simulink model "adaptive_cruise_control_model"  (R2018a)
settings: Solver=ode23t  StartTime=0.0  StopTime=150  MaxStep=0.01  RelTol=1e-3
values from neighbouring files (symbols this model uses):
  ddefault = 5    [linearized_parameters.m]
  K = 0.07536    [linearized_parameters.m]
  rw = 0.3    [linearized_parameters.m]
  tlag = 3    [linearized_parameters.m]
undefined symbols (not defined in the file or in its folder): sigbuilder_block
libraries: simulink x7, dspsigops x1
settings Model: EnablePacing=on  Creator=Saurabh Suman  LastModifiedBy=Saurabh Suman

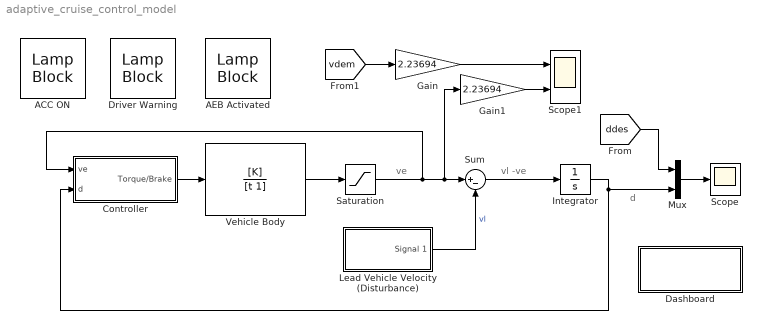
== system adaptive_cruise_control_model ==
  note: d
  note: vl -ve
  note: ve
  ACC ON : LampBlock  WebBlockId=122
  AEB Activated : LampBlock  WebBlockId=120
  Controller : Subsystem
  Dashboard : Subsystem
  Driver Warning : LampBlock  WebBlockId=121
  Gain : Gain  Gain=2.23694
  Gain1 : Gain  Gain=2.23694
  Integrator : Integrator  InitialCondition=100
  Lead Vehicle Velocity (Disturbance) : Subsystem  Tag=STV Subsys  LoadFcn=sigbuilder_block('load');  StartFcn=sigbuilder_block('start');  StopFcn=sigbuilder_block('stop');  ClipboardFcn=sigbuilder_block('clipboard');  mask(Sigbuilder block){tuvar=[0:10]}
      mask help: Simulink:masks:SigbuilderBlock_MD
      mask init:
      | if ~strcmp(get_param(bdroot(gcbh),'SimulationStatus'),'stopped') tuvar = sigbuilder_block('maskInit'); end
      settings: CopyFcn=sigbuilder_block('copy');  DeleteFcn=sigbuilder_block('delete');  ModelCloseFcn=sigbuilder_block('modelClose');  PreSaveFcn=sigbuilder_block('preSave');  PauseFcn=sigbuilder_block('pause');  ContinueFcn=sigbuilder_block('continue');  NameChangeFcn=sigbuilder_block('namechange');  OpenFcn=sigbuilder_block('open',[456.6 167.4 550.8 400.2 ]);  CloseFcn=sigbuilder_block('close');
      mask Display: plot(0, 0, 100, 100,[2, 2, 32, 32, 2], [68, 8, 8, 68, 68],[32, 2], [38, 38], [32, 19, 2],[53, 60, 44], [32, 17, 17, 2],[16, 16, 31, 31]);txt = getActiveGroup(gcbh);text(2, 100, txt,'verticalAlignment', 'top');
  Mux : Mux  Inputs=2
  Saturation : Saturate  UpperLimit=Inf  LowerLimit=0  ZeroCross=off
  Scope : Scope
  Scope1 : Scope  NumInputPorts=2
  Sum : Sum  Inputs=|+-
  Vehicle Body : TransferFcn  Numerator=[K]  Denominator=[t 1]
  wires:
  Lead Vehicle Velocity (Disturbance)/1(Signal 1) -> Sum/2  "vl"
  Saturation/1 -> Controller/1(ve), Gain1/1, Sum/1
  Vehicle Body/1 -> Saturation/1
  Controller/1(Torque/Brake) -> Vehicle Body/1
  Sum/1 -> Integrator/1
  Integrator/1 -> Mux/2, Controller/2(d)
  [ddes] -> Mux/1
  Mux/1 -> Scope/1
  [vdem] -> Gain/1
  Gain/1 -> Scope1/1
  Gain1/1 -> Scope1/2

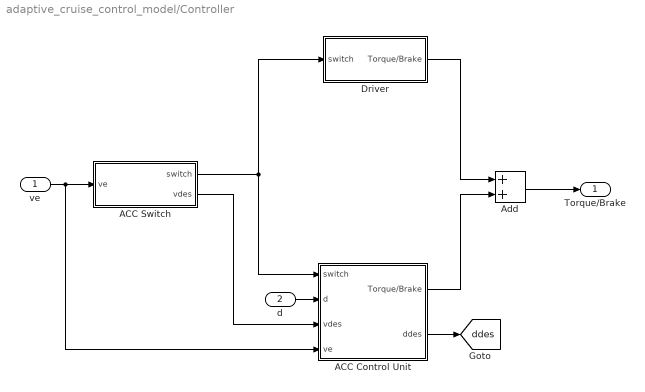
== system adaptive_cruise_control_model/Controller ==
  ve : Inport
  d : Inport  Port=2
  ACC Control Unit : Subsystem
  ACC Switch : Subsystem
  Add : Sum
  Driver : Subsystem
  Torque/Brake : Outport
  tag scope: ddes=global
  wires:
  ve/1 -> ACC Control Unit/4(ve), ACC Switch/1(ve)
  d/1 -> ACC Control Unit/2(d)
  ACC Switch/1(switch) -> Driver/1(switch), ACC Control Unit/1(switch)
  ACC Switch/2(vdes) -> ACC Control Unit/3(vdes)
  ACC Control Unit/1(Torque/Brake) -> Add/2
  Driver/1(Torque/Brake) -> Add/1
  Add/1 -> Torque/Brake/1
  ACC Control Unit/2(ddes) -> [ddes]

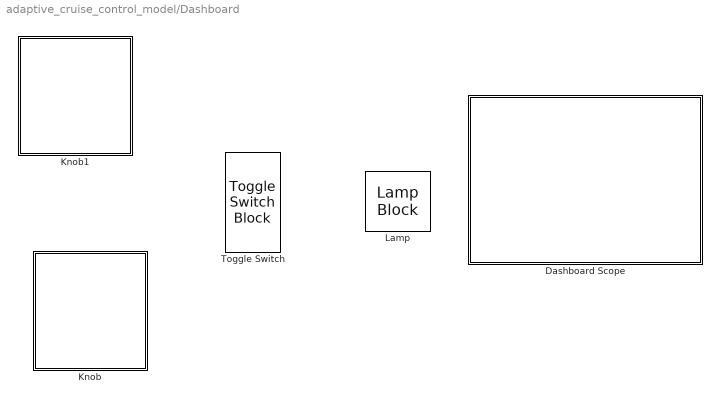
== system adaptive_cruise_control_model/Dashboard ==
  Dashboard Scope : Subsystem  DialogController=hmiCreateDDGDialog  IsWebBlock=on  mask(MWDashboardBlock){webBlockId=a9cadf37-32fc-4d88-93af-27b178824d04, webBlockType=sdiscope, ShowInitialText=on, HMISrcModelName=adaptive_cruise_control_model}
      mask prompts: webBlockId "WebBlock Id"; webBlockType "WebBlock Type"; HMISrcModelName "Source Model"
      mask help: SimulinkHMI:dialogs:HMIScopeDialogDesc
      mask Help: helpview([docroot '/mapfiles/simulink.map'], 'hmi_scope')
      mask Display:
      | if strcmp(get_param(bdroot(gcb),'BlockDiagramType'), 'library')
      |     image([(matlabroot) '/toolbox/simulink/hmi/icons/DashboardScope.png']);
      | end
  Knob : Subsystem  DialogController=hmiCreateDDGDialog  IsWebBlock=on  mask(MWDashboardBlock){webBlockId=72363b14-a3cf-4823-9712-4e9a4279af6e, webBlockType=continuousknob, ShowInLibBrowser=on, ShowInitialText=on, HMISrcModelName=adaptive_cruise_control_model}
      mask prompts: webBlockId "WebBlock Id"; webBlockType "WebBlock Type"; HMISrcModelName "Source Model"
      mask help: SimulinkHMI:dialogs:ContinuousKnobDialogDesc
      mask Help: helpview([docroot '/mapfiles/simulink.map'], 'hmi_knob')
      mask Display:
      | if strcmp(get_param(bdroot(gcb),'BlockDiagramType'), 'library')
      |     image([(matlabroot) '/toolbox/simulink/hmi/icons/ContinuousKnob.png']);
      | end
  Knob1 : Subsystem  DialogController=hmiCreateDDGDialog  IsWebBlock=on  mask(MWDashboardBlock){webBlockId=54317ec1-8d0a-43bc-8178-3813509fb264, webBlockType=continuousknob, ShowInLibBrowser=on, ShowInitialText=on, HMISrcModelName=adaptive_cruise_control_model}
      mask prompts: webBlockId "WebBlock Id"; webBlockType "WebBlock Type"; HMISrcModelName "Source Model"
      mask help: SimulinkHMI:dialogs:ContinuousKnobDialogDesc
      mask Help: helpview([docroot '/mapfiles/simulink.map'], 'hmi_knob')
      mask Display:
      | if strcmp(get_param(bdroot(gcb),'BlockDiagramType'), 'library')
      |     image([(matlabroot) '/toolbox/simulink/hmi/icons/ContinuousKnob.png']);
      | end
  Lamp : LampBlock  WebBlockId=128
  Toggle Switch : ToggleSwitchBlock  WebBlockId=129
      settings: Values={{'Off', 'On'}, [0 1]}

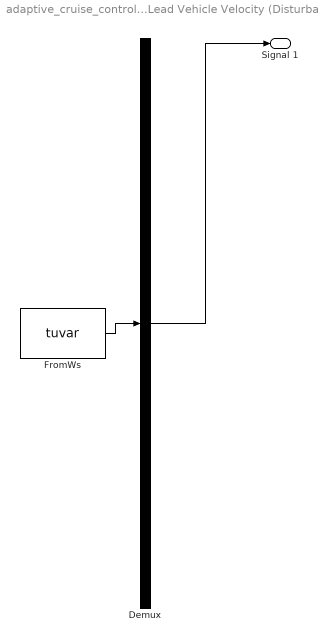
== system adaptive_cruise_control_model/Lead Vehicle Velocity (Disturbance) ==
  Demux : Demux  Tag=STV Demux  Outputs=1
  FromWs : FromWorkspace  Tag=STV FromWs  VariableName=tuvar  SampleTime=0
      SigBuilderData=|
      | common.afterFinalStr = 'Extrapolate'
      | common.sampleTime = 0
      | dataSet(1).timeRange = [0 150]
      | dataSet(1).name = 'Scenario 1'
      | dataSet(2).timeRange = [0 150]
      | dataSet(2).name = 'Scenario 2'
      | dataSet(3).timeRange = [0 150]
      | dataSet(3).name = 'Scenario 3'
      | dataSet(4).timeRange = [0 150]
      | dataSet(4).name = 'Scenario 4'
      | sbobj.Groups(1).Name = 'Scenario 1'
      | sbobj.Groups(1).Signals.Name = 'Signal 1'
      | sbobj.Groups(1).Signals.XData = [0 150]
      | sbobj.Groups(1).Signals.YData = [40 40]
      | sbobj.Groups(1).TimeRange = [0 150]
      | sbobj.Groups(2).Name = 'Scenario 2'
      | sbobj.Groups(2).Signals.Name = 'Signal 1'
      | sbobj.Groups(2).Signals.XData = [0 30 70 80 100 150]
      | sbobj.Groups(2).Signals.YData = [25 25 15 15 30 30]
      | sbobj.Groups(2).TimeRange = [0 150]
      | sbobj.Groups(3).Name = 'Scenario 3'
      | sbobj.Groups(3).Signals.Name = 'Signal 1'
      | sbobj.Groups(3).Signals.XData = [0 30 70 80 100 150]
      | sbobj.Groups(3).Signals.YData = [25 25 15 15 25 25]
      | sbobj.Groups(3).TimeRange = [0 150]
      | sbobj.Groups(4).Name = 'Scenario 4'
      | sbobj.Groups(4).Signals.Name = 'Signal 1'
      | sbobj.Groups(4).Signals.XData = [0 30 70 80 100 150]
      | sbobj.Groups(4).Signals.YData = [25 25 0 0 25 25]
      | sbobj.Groups(4).TimeRange = [0 150]
  Signal 1 : Outport  Tag=STV Outport
  wires:
  Demux/1 -> Signal 1/1
  FromWs/1 -> Demux/1

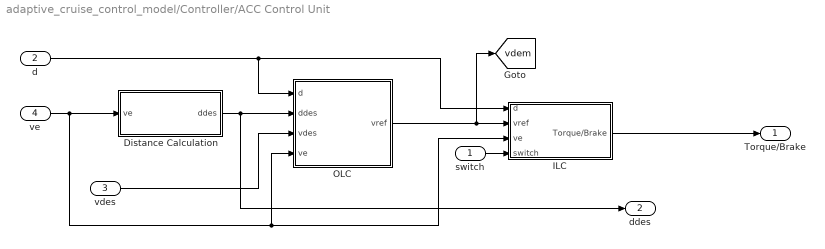
== system adaptive_cruise_control_model/Controller/ACC Control Unit ==
  switch : Inport
  d : Inport  Port=2
  vdes : Inport  Port=3
  ve : Inport  Port=4
  Distance Calculation : Subsystem
  ILC : Subsystem
  OLC : Subsystem
  Torque/Brake : Outport
  ddes : Outport  Port=2
  tag scope: vdem=global
  wires:
  OLC/1(vref) -> [vdem], ILC/2(vref)
  d/1 -> ILC/1(d), OLC/1(d)
  ve/1 -> ILC/3(ve), OLC/4(ve), Distance Calculation/1(ve)
  Distance Calculation/1(ddes) -> ddes/1, OLC/2(ddes)
  vdes/1 -> OLC/3(vdes)
  switch/1 -> ILC/4(switch)
  ILC/1(Torque/Brake) -> Torque/Brake/1

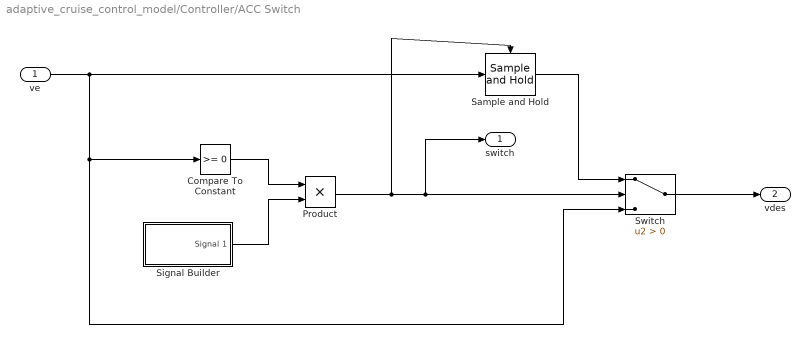
== system adaptive_cruise_control_model/Controller/ACC Switch ==
  ve : Inport
  Compare To Constant : simulink/Logic and Bit Operations/Compare To Constant  relop=>=  const=0  OutDataTypeStr=boolean
  Product : Product
  Sample and Hold : dspsigops/Sample and Hold  trig=Rising edge  initCond=0  latchinput=off
  Signal Builder : Subsystem  Tag=STV Subsys  LoadFcn=sigbuilder_block('load');  StartFcn=sigbuilder_block('start');  StopFcn=sigbuilder_block('stop');  ClipboardFcn=sigbuilder_block('clipboard');  mask(Sigbuilder block){tuvar=[0:10]}
      mask help: Simulink:masks:SigbuilderBlock_MD
      mask init:
      | if ~strcmp(get_param(bdroot(gcbh),'SimulationStatus'),'stopped') tuvar = sigbuilder_block('maskInit'); end
      settings: CopyFcn=sigbuilder_block('copy');  DeleteFcn=sigbuilder_block('delete');  ModelCloseFcn=sigbuilder_block('modelClose');  PreSaveFcn=sigbuilder_block('preSave');  PauseFcn=sigbuilder_block('pause');  ContinueFcn=sigbuilder_block('continue');  NameChangeFcn=sigbuilder_block('namechange');  OpenFcn=sigbuilder_block('open',[453.6 160.2 550.8 400.2 ]);  CloseFcn=sigbuilder_block('close');
      mask Display: plot(0, 0, 100, 100,[2, 2, 32, 32, 2], [68, 8, 8, 68, 68],[32, 2], [38, 38], [32, 19, 2],[53, 60, 44], [32, 17, 17, 2],[16, 16, 31, 31]);txt = getActiveGroup(gcbh);text(2, 100, txt,'verticalAlignment', 'top');
  Switch : Switch  Criteria=u2 > Threshold
  switch : Outport
  vdes : Outport  Port=2
  wires:
  Sample and Hold/1 -> Switch/1
  Switch/1 -> vdes/1
  Compare To Constant/1 -> Product/1
  Signal Builder/1(Signal 1) -> Product/2
  ve/1 -> Compare To Constant/1, Switch/3, Sample and Hold/1
  Product/1 -> Sample and Hold/Trigger, switch/1, Switch/2

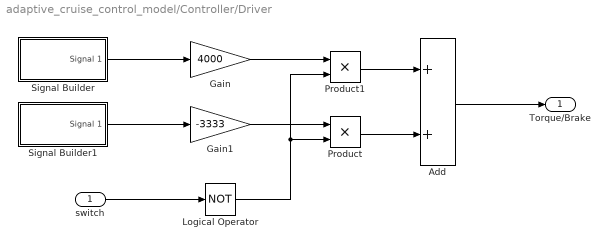
== system adaptive_cruise_control_model/Controller/Driver ==
  switch : Inport
  Add : Sum
  Gain : Gain  Gain=4000
  Gain1 : Gain  Gain=-3333
  Logical Operator : Logic  Operator=NOT  AllPortsSameDT=off  OutDataTypeStr=boolean
  Product : Product
  Product1 : Product
  Signal Builder : Subsystem  Tag=STV Subsys  LoadFcn=sigbuilder_block('load');  StartFcn=sigbuilder_block('start');  StopFcn=sigbuilder_block('stop');  ClipboardFcn=sigbuilder_block('clipboard');  mask(Sigbuilder block){tuvar=[0:10]}
      mask help: Simulink:masks:SigbuilderBlock_MD
      mask init:
      | if ~strcmp(get_param(bdroot(gcbh),'SimulationStatus'),'stopped') tuvar = sigbuilder_block('maskInit'); end
      settings: CopyFcn=sigbuilder_block('copy');  DeleteFcn=sigbuilder_block('delete');  ModelCloseFcn=sigbuilder_block('modelClose');  PreSaveFcn=sigbuilder_block('preSave');  PauseFcn=sigbuilder_block('pause');  ContinueFcn=sigbuilder_block('continue');  NameChangeFcn=sigbuilder_block('namechange');  OpenFcn=sigbuilder_block('open',[470.4 157.8 550.8 400.2 ]);  CloseFcn=sigbuilder_block('close');
      mask Display: plot(0, 0, 100, 100,[2, 2, 32, 32, 2], [68, 8, 8, 68, 68],[32, 2], [38, 38], [32, 19, 2],[53, 60, 44], [32, 17, 17, 2],[16, 16, 31, 31]);txt = getActiveGroup(gcbh);text(2, 100, txt,'verticalAlignment', 'top');
  Signal Builder1 : Subsystem  Tag=STV Subsys  LoadFcn=sigbuilder_block('load');  StartFcn=sigbuilder_block('start');  StopFcn=sigbuilder_block('stop');  ClipboardFcn=sigbuilder_block('clipboard');  mask(Sigbuilder block){tuvar=[0:10]}
      mask help: Simulink:masks:SigbuilderBlock_MD
      mask init:
      | if ~strcmp(get_param(bdroot(gcbh),'SimulationStatus'),'stopped') tuvar = sigbuilder_block('maskInit'); end
      settings: CopyFcn=sigbuilder_block('copy');  DeleteFcn=sigbuilder_block('delete');  ModelCloseFcn=sigbuilder_block('modelClose');  PreSaveFcn=sigbuilder_block('preSave');  PauseFcn=sigbuilder_block('pause');  ContinueFcn=sigbuilder_block('continue');  NameChangeFcn=sigbuilder_block('namechange');  OpenFcn=sigbuilder_block('open',[470.4 157.8 550.8 400.2 ]);  CloseFcn=sigbuilder_block('close');
      mask Display: plot(0, 0, 100, 100,[2, 2, 32, 32, 2], [68, 8, 8, 68, 68],[32, 2], [38, 38], [32, 19, 2],[53, 60, 44], [32, 17, 17, 2],[16, 16, 31, 31]);txt = getActiveGroup(gcbh);text(2, 100, txt,'verticalAlignment', 'top');
  Torque/Brake : Outport
  wires:
  Signal Builder/1(Signal 1) -> Gain/1
  Signal Builder1/1(Signal 1) -> Gain1/1
  switch/1 -> Logical Operator/1
  Gain/1 -> Product1/1
  Gain1/1 -> Product/1
  Logical Operator/1 -> Product/2, Product1/2
  Product1/1 -> Add/1
  Product/1 -> Add/2
  Add/1 -> Torque/Brake/1

== system adaptive_cruise_control_model/Dashboard/Dashboard Scope ==

== system adaptive_cruise_control_model/Dashboard/Knob ==

== system adaptive_cruise_control_model/Dashboard/Knob1 ==

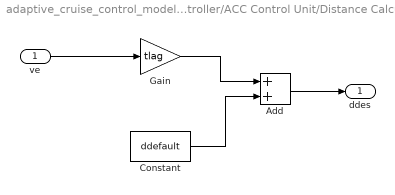
== system adaptive_cruise_control_model/Controller/ACC Control Unit/Distance Calculation ==
  ve : Inport
  Add : Sum
  Constant : Constant  Value=ddefault
  Gain : Gain  Gain=tlag
  ddes : Outport
  wires:
  ve/1 -> Gain/1
  Gain/1 -> Add/1
  Constant/1 -> Add/2
  Add/1 -> ddes/1

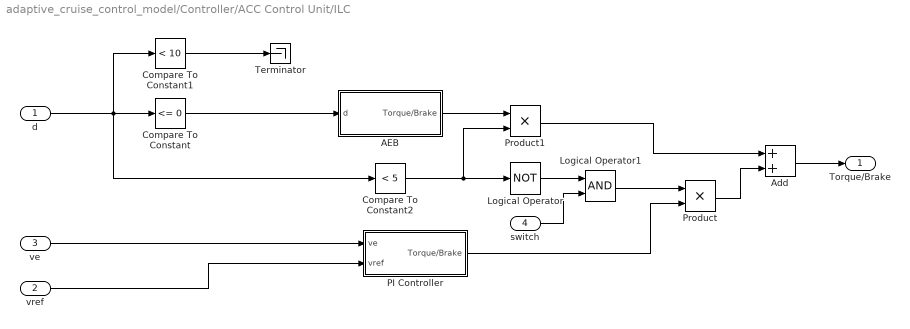
== system adaptive_cruise_control_model/Controller/ACC Control Unit/ILC ==
  d : Inport
  vref : Inport  Port=2
  ve : Inport  Port=3
  switch : Inport  Port=4
  AEB : Subsystem
  Add : Sum
  Compare To Constant : simulink/Logic and Bit Operations/Compare To Constant  relop=<=  const=0  OutDataTypeStr=boolean
  Compare To Constant1 : simulink/Logic and Bit Operations/Compare To Constant  relop=<  const=10  OutDataTypeStr=boolean
  Compare To Constant2 : simulink/Logic and Bit Operations/Compare To Constant  relop=<  const=5  OutDataTypeStr=boolean
  Logical Operator : Logic  Operator=NOT  AllPortsSameDT=off  OutDataTypeStr=boolean
  Logical Operator1 : Logic  AllPortsSameDT=off  OutDataTypeStr=boolean
  PI Controller : Subsystem
  Product : Product
  Product1 : Product
  Terminator : Terminator
  Torque/Brake : Outport
  wires:
  Add/1 -> Torque/Brake/1
  Logical Operator1/1 -> Product/1
  d/1 -> Compare To Constant1/1, Compare To Constant2/1, Compare To Constant/1
  ve/1 -> PI Controller/1(ve)
  vref/1 -> PI Controller/2(vref)
  Compare To Constant1/1 -> Terminator/1
  Compare To Constant/1 -> AEB/1(d)
  Compare To Constant2/1 -> Product1/2, Logical Operator/1
  AEB/1(Torque/Brake) -> Product1/1
  Logical Operator/1 -> Logical Operator1/1
  switch/1 -> Logical Operator1/2
  PI Controller/1(Torque/Brake) -> Product/2
  Product/1 -> Add/2
  Product1/1 -> Add/1

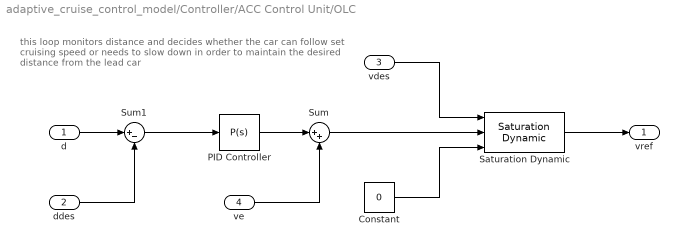
== system adaptive_cruise_control_model/Controller/ACC Control Unit/OLC ==
  note: this loop monitors distance and decides whether the car can follow set cruising speed or needs to slow down in order to maintain the desired distance from the lead car
  d : Inport
  ddes : Inport  Port=2
  vdes : Inport  Port=3
  ve : Inport  Port=4
  Constant : Constant  Value=0
  PID Controller : simulink/Continuous/PID Controller  Controller=P  TimeDomain=Continuous-time  SampleTime=-1  IntegratorMethod=Forward Euler  FilterMethod=Forward Euler  Form=Parallel  UseFilter=on  ControllerParametersSource=internal  P=5  I=1  D=0  N=100  InitialConditionSource=internal  InitialConditionForIntegrator=0  InitialConditionForFilter=0  ExternalReset=none  LimitOutput=off  UpperSaturationLimit=inf  LowerSaturationLimit=-inf  LinearizeAsGain=on  AntiWindupMode=none  Kb=1  TrackingMode=off  Kt=1  PParamMin=[]  PParamMax=[]  IParamMin=[]  IParamMax=[]  DParamMin=[]  DParamMax=[]  NParamMin=[]  NParamMax=[]  KbParamMin=[]  KbParamMax=[]  KtParamMin=[]  KtParamMax=[]  POutMin=[]  POutMax=[]  IOutMin=[]  IOutMax=[]  DOutMin=[]  DOutMax=[]  NOutMin=[]  NOutMax=[]  KbOutMin=[]  KbOutMax=[]  KtOutMin=[]  KtOutMax=[]  IntegratorOutMin=[]  IntegratorOutMax=[]  FilterOutMin=[]  FilterOutMax=[]  SumOutMin=[]  SumOutMax=[]  SumI1OutMin=[]  SumI1OutMax=[]  SumI2OutMin=[]  SumI2OutMax=[]  SumI3OutMin=[]  SumI3OutMax=[]  SumDOutMin=[]  SumDOutMax=[]  SaturationOutMin=[]  SaturationOutMax=[]  IntegratorContinuousStateAttributes=''  IntegratorStateMustResolveToSignalObject=off  IntegratorRTWStateStorageClass=Auto  FilterContinuousStateAttributes=''  FilterStateMustResolveToSignalObject=off  FilterRTWStateStorageClass=Auto  DifferentiatorICPrevScaledInput=0  DifferentiatorOutMin=[]  DifferentiatorOutMax=[]  FilterDiffOutCoefMin=[]  FilterDiffOutCoefMax=[]  SumDenOutMin=[]  SumDenOutMax=[]  SumNumOutMin=[]  SumNumOutMax=[]  ReciprocalOutMin=[]  ReciprocalOutMax=[]  DivideOutMin=[]  DivideOutMax=[]  TunerSelectOption=Transfer Function Based (PID Tuner App)
  Saturation Dynamic : simulink/Discontinuities/Saturation Dynamic  OutMin=[]  OutMax=[]  OutDataTypeStr=Inherit: Same as second input  OutDataType=fixdt(1, 16)  OutScaling=2^-10  DoSatur=off
  Sum : Sum  Inputs=|++
  Sum1 : Sum  Inputs=|+-
  vref : Outport
  wires:
  d/1 -> Sum1/1
  PID Controller/1 -> Sum/1
  Sum1/1 -> PID Controller/1
  ddes/1 -> Sum1/2
  ve/1 -> Sum/2
  vdes/1 -> Saturation Dynamic/1
  Constant/1 -> Saturation Dynamic/3
  Sum/1 -> Saturation Dynamic/2
  Saturation Dynamic/1 -> vref/1

== system adaptive_cruise_control_model/Controller/ACC Switch/Signal Builder ==
  Demux : Demux  Tag=STV Demux  Outputs=1
  FromWs : FromWorkspace  Tag=STV FromWs  VariableName=tuvar  SampleTime=0
      SigBuilderData=|
      | common.afterFinalStr = 'Extrapolate'
      | common.sampleTime = 0
      | dataSet(1).timeRange = [0 150]
      | dataSet(1).name = 'Scenario 1'
      | dataSet(2).timeRange = [0 150]
      | dataSet(2).name = 'Scenario 2-4'
      | sbobj.Groups(1).Name = 'Scenario 1'
      | sbobj.Groups(1).Signals.Name = 'Signal 1'
      | sbobj.Groups(1).Signals.XData = [0 10 10 80 80 150]
      | sbobj.Groups(1).Signals.YData = [0 0 1 1 0 0]
      | sbobj.Groups(1).TimeRange = [0 150]
      | sbobj.Groups(2).Name = 'Scenario 2-4'
      | sbobj.Groups(2).Signals.Name = 'Signal 1'
      | sbobj.Groups(2).Signals.XData = [0 10 10 150]
      | sbobj.Groups(2).Signals.YData = [0 0 1 1]
      | sbobj.Groups(2).TimeRange = [0 150]
  Signal 1 : Outport  Tag=STV Outport
  wires:
  Demux/1 -> Signal 1/1
  FromWs/1 -> Demux/1

== system adaptive_cruise_control_model/Controller/Driver/Signal Builder ==
  Demux : Demux  Tag=STV Demux  Outputs=1
  FromWs : FromWorkspace  Tag=STV FromWs  VariableName=tuvar  SampleTime=0
      SigBuilderData=|
      | common.afterFinalStr = 'Extrapolate'
      | common.sampleTime = 0
      | dataSet(1).timeRange = [0 150]
      | dataSet(1).name = 'Scenario 1'
      | dataSet(2).timeRange = [0 150]
      | dataSet(2).name = 'Scenario 2-4'
      | sbobj.Groups(1).Name = 'Scenario 1'
      | sbobj.Groups(1).Signals.Name = 'Signal 1'
      | sbobj.Groups(1).Signals.XData = [0 10 10 100 100 120 120 150]
      | sbobj.Groups(1).Signals.YData = [0.7 0.7 0 0 0.3 0.3 0 0]
      | sbobj.Groups(1).TimeRange = [0 150]
      | sbobj.Groups(2).Name = 'Scenario 2-4'
      | sbobj.Groups(2).Signals.Name = 'Signal 1'
      | sbobj.Groups(2).Signals.XData = [0 10 10 150]
      | sbobj.Groups(2).Signals.YData = [0.7 0.7 0 0]
      | sbobj.Groups(2).TimeRange = [0 150]
  Signal 1 : Outport  Tag=STV Outport
  wires:
  Demux/1 -> Signal 1/1
  FromWs/1 -> Demux/1

== system adaptive_cruise_control_model/Controller/Driver/Signal Builder1 ==
  Demux : Demux  Tag=STV Demux  Outputs=1
  FromWs : FromWorkspace  Tag=STV FromWs  VariableName=tuvar  SampleTime=0
      SigBuilderData=|
      | common.afterFinalStr = 'Extrapolate'
      | common.sampleTime = 0
      | dataSet(1).timeRange = [0 150]
      | dataSet(1).name = 'Scenario 1'
      | dataSet(2).timeRange = [0 150]
      | dataSet(2).name = 'Scenario 2-4'
      | sbobj.Groups(1).Name = 'Scenario 1'
      | sbobj.Groups(1).Signals.Name = 'Signal 1'
      | sbobj.Groups(1).Signals.XData = [0 80 80 100 100 120 120 150]
      | sbobj.Groups(1).Signals.YData = [0 0 0.1 0.1 0 0 0.05 0.05]
      | sbobj.Groups(1).TimeRange = [0 150]
      | sbobj.Groups(2).Name = 'Scenario 2-4'
      | sbobj.Groups(2).Signals.Name = 'Signal 1'
      | sbobj.Groups(2).Signals.XData = [0 150]
      | sbobj.Groups(2).Signals.YData = [0 0]
      | sbobj.Groups(2).TimeRange = [0 150]
  Signal 1 : Outport  Tag=STV Outport
  wires:
  Demux/1 -> Signal 1/1
  FromWs/1 -> Demux/1

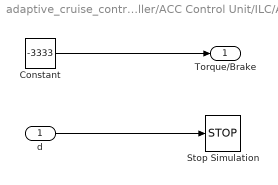
== system adaptive_cruise_control_model/Controller/ACC Control Unit/ILC/AEB ==
  d : Inport
  Constant : Constant  Value=-3333
  Stop Simulation : Stop
  Torque/Brake : Outport
  wires:
  d/1 -> Stop Simulation/1
  Constant/1 -> Torque/Brake/1

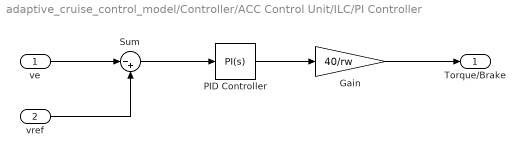
== system adaptive_cruise_control_model/Controller/ACC Control Unit/ILC/PI Controller ==
  ve : Inport
  vref : Inport  Port=2
  Gain : Gain  Gain=40/rw
  PID Controller : simulink/Continuous/PID Controller  Controller=PI  TimeDomain=Continuous-time  SampleTime=-1  IntegratorMethod=Forward Euler  FilterMethod=Forward Euler  Form=Parallel  UseFilter=on  ControllerParametersSource=internal  P=10  I=50  D=0  N=100  InitialConditionSource=internal  InitialConditionForIntegrator=0  InitialConditionForFilter=0  ExternalReset=none  LimitOutput=off  UpperSaturationLimit=inf  LowerSaturationLimit=-inf  LinearizeAsGain=on  AntiWindupMode=none  Kb=1  TrackingMode=off  Kt=1  PParamMin=[]  PParamMax=[]  IParamMin=[]  IParamMax=[]  DParamMin=[]  DParamMax=[]  NParamMin=[]  NParamMax=[]  KbParamMin=[]  KbParamMax=[]  KtParamMin=[]  KtParamMax=[]  POutMin=[]  POutMax=[]  IOutMin=[]  IOutMax=[]  DOutMin=[]  DOutMax=[]  NOutMin=[]  NOutMax=[]  KbOutMin=[]  KbOutMax=[]  KtOutMin=[]  KtOutMax=[]  IntegratorOutMin=[]  IntegratorOutMax=[]  FilterOutMin=[]  FilterOutMax=[]  SumOutMin=[]  SumOutMax=[]  SumI1OutMin=[]  SumI1OutMax=[]  SumI2OutMin=[]  SumI2OutMax=[]  SumI3OutMin=[]  SumI3OutMax=[]  SumDOutMin=[]  SumDOutMax=[]  SaturationOutMin=[]  SaturationOutMax=[]  IntegratorContinuousStateAttributes=''  IntegratorStateMustResolveToSignalObject=off  IntegratorRTWStateStorageClass=Auto  FilterContinuousStateAttributes=''  FilterStateMustResolveToSignalObject=off  FilterRTWStateStorageClass=Auto  DifferentiatorICPrevScaledInput=0  DifferentiatorOutMin=[]  DifferentiatorOutMax=[]  FilterDiffOutCoefMin=[]  FilterDiffOutCoefMax=[]  SumDenOutMin=[]  SumDenOutMax=[]  SumNumOutMin=[]  SumNumOutMax=[]  ReciprocalOutMin=[]  ReciprocalOutMax=[]  DivideOutMin=[]  DivideOutMax=[]  TunerSelectOption=Transfer Function Based (PID Tuner App)
  Sum : Sum  Inputs=|-+
  Torque/Brake : Outport
  wires:
  Gain/1 -> Torque/Brake/1
  PID Controller/1 -> Gain/1
  Sum/1 -> PID Controller/1
  ve/1 -> Sum/1
  vref/1 -> Sum/2
